simulink model "Experiment_1_cs"  (Simulink 8.4)
settings: Solver=ode5  SolverMode=SingleTasking  StartTime=0.0  StopTime=inf  FixedStep=1/100  RelTol=1e-3
PreLoadFcn:
  | mbxruntime.callbacks.PreLoadFcn(bdroot);
PostLoadFcn:
  | mbxruntime.callbacks.PostLoadFcn(bdroot);
InitFcn:
  | mbxruntime.callbacks.InitFcn(bdroot);
StartFcn:
  | mbxruntime.callbacks.StartFcn(bdroot);
StopFcn:
  | mbxruntime.callbacks.StopFcn(bdroot);
undefined symbols (not defined in the file or in its folder): dfreq, gray, Rec, SDTV, strel
libraries: simulink x42, PreScanSimulinkLibrary x17, visiontextngfix x15, simulink_extras x12, visionconversions x3, PreScanUsefulBlocks x3, visionsinks x2, visionstatistics x1, visionmorphops x1, visionanalysis x1, simulink_need_slupdate x1
(part 2 of 8)

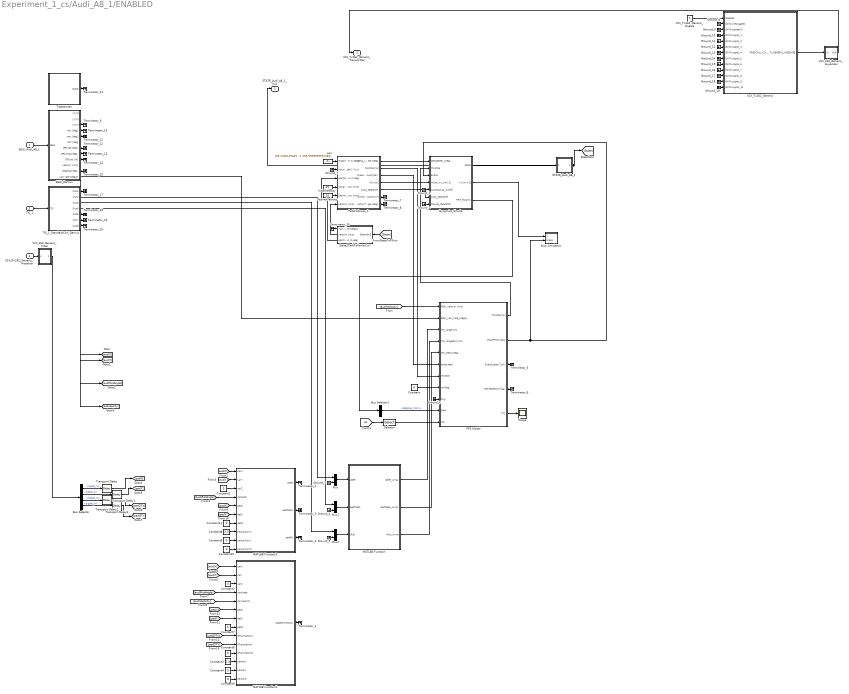
== system Experiment_1_cs/Audi_A8_1/ENABLED ==
  SELF_Audi_A8_1 : Inport  Tag=inport/SelfPort  OutDataTypeStr=Bus: PRESCAN_SELFSENSORDATA  PortDimensions=1  SampleTime=1/100  BusOutputAsStruct=on
  TIS_1 : Inport  Tag=inport/TIS  Port=2  OutDataTypeStr=Bus: PRESCAN_SCANNERSENSOR_MESSAGE  PortDimensions=1  SampleTime=1/50  BusOutputAsStruct=on
  V2X_Rx262_Generic_Receiver : Inport  Tag=inport/plugin/sfun_V2X_Generic_Receiver  Port=3  BusOutputAsStruct=on
  Bus Selector : BusSelector  OutputSignals=DATA.signal_1,DATA.signal_2,DATA.signal_3,DATA.signal_4
  Bus Selector1 : BusSelector  OutputSignals=NEngine_[rpm]
  Constant{,1..2,4..7,9..11} (10 alike) : Constant  Value=0
  Constant3 : Constant  Value=2.3
  Constant8 : Constant  Value=2.3
  DesiredVelocity : Constant  Tag=DesiredVelocity  Value=15
  Dynamics_Simple : Subsystem  Tag=Simple_Vehicle_Dynamics  mask(PreScan Block: Simple Dynamics){Migrate=on, TimeStep=1/100, ComputationMode=Continuous_Time}
      mask prompts: Migrate "Migrate. During migration this block will be replaced by a newer one."; TimeStep "Auto assigned: Time Step [s]"; ComputationMode "Computation mode:"
      mask help:
      | The Simple Dynamics Model is selected in the GUI to simulate vehicle dynamics behavior.
      |
      | The Simple Dynamics Model is completely open to the user. The parameters of this model can be set in the Simple Dynamics dialog in the GUI.
      |
      | For more information, please click Help.
      mask init:
      | p = SimpleDyn_pars;
      settings: DeleteFcn=PreScanBlockDeleteFcn;
      mask Help: eval('openHelp(220)')
      mask Display:
      | image(imread('SimpleDyn.png'))
      | port_label('input', 1, '{\delta}_S_t_ _e_e_r [deg]','texmode','on')
      | port_label('input', 2, 'Throttle [%]')
      | port_label('input', 3, 'Brake Pres [bar]')
      | port_label('input', 4, 'V_0 [ms-1]','texmode','on')
      | port_label('input', 5, 'Auto=[0]/Manual=[1]')
      | port_label('input', 6, 'Auto_GearShift')
      | port_label('input', 7, 'Manual_GearShift')
      | port_label('output', 1, 'State')
      | port_label('output', 2, 'Vx [ms-1]')
      | port_label('output', 3, 'Perf Params')
  Ground_{1..19} (19 alike) : Ground
  InitialVelocity : Constant  Tag=InitialVelocity  Value=15
  MATLAB Function : MATLAB Function  TreatAsAtomicUnit=on
  MATLAB Function1 : MATLAB Function  TreatAsAtomicUnit=on
  MATLAB Function2 : MATLAB Function  TreatAsAtomicUnit=on
  Mux : Mux  Inputs=2
  Mux1 : Mux  Inputs=2
  Mux2 : Mux  Inputs=2
  PPS Model : Subsystem  mask(PPS Model){MaxSpeed=70, MaxBrakePressure=150, BrakeDelay=100, LaneWidth=3.5, TISMaxRange=40, TISMaxTheta=60, TISfreq=25, TISdet=32, Camfreq=50, Mainfreq=100, DisplaySwitch=on, DisplayFreq=25, RadarSwitch=on, RadarFreq=25}
      mask prompts: MaxSpeed "Vehicle cut-off speed [km/h]"; MaxBrakePressure "Maximum value of braking pressure available [bar]"; BrakeDelay "Braking system delay [ms]"; LaneWidth "Lane width [m]"; TISMaxRange "TIS maximum range [m]"; TISMaxTheta "TIS maximum theta [deg]"; TISfreq "TIS frequency [Hz]"; TISdet "Max. number of Radar detected objects [-]"; Camfreq "Camera frequency [Hz]"; Mainfreq "Compilation sheet frequency [Hz]"; DisplaySwitch "Show EGO parameters visualization"; DisplayFreq "EGO parameters visualization frequency [Hz]"; RadarSwitch "Show radar visualization"; RadarFreq "Radar frequency [Hz]"
      mask help: PreScan Experiment and Pedestrian Protection System parameters
      mask Help: eval('openHelp(8130)')
      mask Callback DisplaySwitch:
      | en = get_param(gcb,'MaskEnables');
      | switch get_param(gcb, 'DisplaySwitch')
      |     case 'off'
      |         en{12} = 'off';
      |     case 'on'
      |         en{12} = 'on';
      | end
      | set_param(gcb,'MaskEnables',en);
      mask Callback RadarSwitch:
      | en = get_param(gcb,'MaskEnables');
      | switch get_param(gcb, 'RadarSwitch')
      |     case 'off'
      |         en{14} = 'off';
      |     case 'on'
      |         en{14} = 'on';
      | end
      | set_param(gcb,'MaskEnables',en);
  PathFollower_1 : Subsystem  Tag=pathFollower  mask(PreScan Block: Path Follower){Migrate=on, FileName='Trajectory_2.mat', TunableSteeringGain=1, XShifting_wrt_COG=0}
      mask prompts: Migrate "Migrate. During migration this block will be replaced by a newer one."; FileName "Trajectory Name"; TunableSteeringGain "TunableSteeringGain [-]"; XShifting_wrt_COG "XShifting_wrt_COG [m]"
      mask help:
      | The Path Follower Model is selected in the GUI to simulate driver behavior.
      |
      | For more information, please click Help.
      mask init:
      | load(['trajectories/',eval(FileName)])
      | traject=trajectory';
      | 
      | Traj_x=traject(:,2);
      | Traj_y=traject(:,3);
      | Traj_z=traject(:,4);
      | Traj_vx=traject(:,8);
      | Traj_vy=traject(:,9);
      | Traj_vz=traject(:,10);
      mask Help: eval('openHelp(232)')
  SELF_Demux : Subsystem  Tag=demux/SelfPort  mask(PreScan Demux Block:){}
      mask help:
      | The SELF port shows (state) information of the actor itself. The outputs are position in the experiment's axis system and the GPS coordinates, and the object's absolute velocity and compass heading.
      |
      | For more information, please click Help.
      settings: DeleteFcn=PreScanBlockDeleteFcn;
      mask Help: eval('openHelp(462)')
      mask Display:
      | port_label('output',1,'x [m]')
      | port_label('output',2,'y [m]')
      | port_label('output',3,'z [m]','texmode','on')
      | port_label('output',4,'Rotx [deg]','texmode','on')
      | port_label('output',5,'Roty [deg]','texmode','on')
      | port_label('output',6,'Rotz [deg]','texmode','on')
      | port_label('output',7,'GPS lat [deg]','texmode','on')
      | port_label('output',8,'GPS long [deg]','texmode','on')
      | port_label('output',9,'GPS alt [m]','texmode','on')
      | port_label('output',10,'Velocity [m/s]')
      | port_label('output',11,'Heading [deg]')
      | port_label('output',12,'Yaw rate [deg/s]')
  STATE_Audi_A8_1 : Subsystem  Tag=mux/StatePort  Priority=0  LoadFcn=load PrescanStateActuatorData  mask(PreScan Sink Block: State){x0=99.430015563964844, y0=124.71636199951172, z0=0.55, Roll0=0, Pitch0=0, Yaw0=359.9999999997284, TimeStep=1/100}
      mask prompts: x0 "Ini x-position VEHICLE wrt GLOBAL axis system [m]"; y0 "Ini y-position VEHICLE wrt GLOBAL axis system [m]"; z0 "Ini z-position VEHICLE wrt GLOBAL axis system [m]"; Roll0 "Ini roll-angle BODY wrt VEHICLE axis system [deg]"; Pitch0 "Ini pitch-angle BODY wrt VEHICLE axis system [deg]"; Yaw0 "Ini yaw-angle VEHICLE wrt GLOBAL axis system [deg]"; TimeStep "Auto-Assigned: Upload Period [s]"
      mask help:
      | The Actor State contains a vector signal of size (9x1), containing the following signals:
      |
      | -  Position                  (x,y,z)                                     [m]
      | -  Velocity                  (vx,vy,vz)                               [m/s]
      | -  Angles                    (Roll, Pitch, Yaw)                   [rad]
      |
      | The Actor state is defined in the global axis system.
      | The state is superponed on the Initial position defined in the GUI.
      |
      | For more information, please click Help.
      settings: DeleteFcn=PreScanBlockDeleteFcn;
      mask Help: eval('openHelp(222)')
      mask Display: image(imread('State.png'))
  Scope : Scope
  Selector : Selector  InputPortWidth=5
  State2PathFollowerCnv : Subsystem  Tag=State2PFConnection/cnv
  Stop simulation : Subsystem
  TIS_1_StandardCoh_Demux : Subsystem  Tag=demux/TIS/StandardCoh  TreatAsAtomicUnit=on  mask(PreScan Demux Block: TIS){MAXMESSAGES=1}
      mask prompts: MAXMESSAGES "Number of Objects"
      mask Help: eval('openHelp(449)')
      mask Display:
      | port_label('input',1,'TIS')
      | port_label('output',1,'Beam ID [-]')
      | port_label('output',2,'Range [m]')
      | port_label('output',3,'DopplerVelocity [m/s]')
      | port_label('output',4,'{\theta} [deg]','texmode','on')
      | port_label('output',5,'{\phi} [deg]','texmode','on')
      | port_label('output',6,'Target ID [-]','texmode','on')
      | port_label('output',7,'TIS Data','texmode','on')
  Terminator_{1..21} (21 alike) : Terminator
  Trajectories : Subsystem  Tag=Trajectories  mask(PreScan Source Block: Trajectories){}
      mask help:
      | The Trajectory block contains the trajectories defined in the PreScan Experiment Editor. The output of the trajectory block is the (vehicle) State.
      |
      | For more information, please click Help.
      settings: DeleteFcn=PreScanBlockDeleteFcn;
      mask Help: eval('openHelp(312)')
      mask Display: image(imread('Trajectory.png'));
  Transport Delay{,1..3} (4 alike) : TransportDelay  DelayTime=0
  V2X_262_Generic_Expander : Subsystem  LoadFcn=addpath .\V2XPlugin; V2Xbusses;
  V2X_262_Generic_Filter : Subsystem
      mask Display: disp('[1]');
  V2X_Tx262_Generic : Subsystem
  V2X_Tx262_Generic_Enable : Constant  OutDataTypeStr=Inherit: Inherit via back propagation
  pos : Constant  Tag=pos  Value=[99.430015563964844 124.71636199951172 359.9999999997284]
  STATE_Audi_A8_1_bus : Outport  Tag=outport/StatePort  OutDataTypeStr=Bus: PRESCAN_STATEACTUATORDATA  PortDimensions=1  SampleTime=1/100
  V2X_Tx262_Generic_Transmitter : Outport  Tag=outport/plugin/sfun_V2X_Generic_Transmitter  Port=2
  wires:
  Dynamics_Simple/3(Perf_Params) -> Bus Selector1/1
  SELF_Demux/12(yaw rate [deg/s]) -> PPS Model/2(EGO_yaw_rate_[deg/s])
  TIS_1_StandardCoh_Demux/2(Out2) -> Mux/1
  TIS_1_StandardCoh_Demux/3(Out3) -> Mux2/1
  TIS_1_StandardCoh_Demux/4(Out4) -> Mux1/1
  [audiX] -> MATLAB Function2/1(carX)
  [audiY] -> MATLAB Function2/2(carY)
  Constant1/1 -> MATLAB Function2/3(carZ)
  [audiRotAngle] -> MATLAB Function2/4(carRotZ)
  [audiX] -> MATLAB Function1/1(carX)
  [audiY] -> MATLAB Function1/2(carY)
  Constant2/1 -> MATLAB Function1/3(carZ)
  [audiRotAngle] -> MATLAB Function1/4(carAngle)
  [audiVelocity] -> MATLAB Function1/5(carVelocity)
  Constant3/1 -> MATLAB Function1/12(sensorX)
  Constant4/1 -> MATLAB Function1/13(sensorY)
  Constant5/1 -> MATLAB Function1/14(sensorZ)
  Constant6/1 -> MATLAB Function1/11(dTranslationZ)
  Constant7/1 -> MATLAB Function1/8(pedZ)
  Constant8/1 -> MATLAB Function2/8(sensorCorrX)
  Constant9/1 -> MATLAB Function2/9(sensorCorrY)
  Constant10/1 -> MATLAB Function2/10(sensorCorrZ)
  Constant11/1 -> MATLAB Function2/7(pedZ)
  [pedX] -> MATLAB Function2/5(pedX)
  [pedY] -> MATLAB Function2/6(pedY)
  [pedX] -> MATLAB Function1/6(pedX)
  [pedY] -> MATLAB Function1/7(pedY)
  [pedDTX] -> MATLAB Function1/9(dTranslationX)
  [pedDTY] -> MATLAB Function1/10(dTranslationY)
  SELF_Demux/1(x [m]) -> [audiX]
  SELF_Demux/2(y [m]) -> [audiY]
  SELF_Demux/6(rotz [deg]) -> [audiRotAngle]
  SELF_Demux/10(velocity [m/s]) -> [audiVelocity]
  [audiVelocity] -> PPS Model/1(EGO_velocity [m/s])
  Bus Selector1/1 -> PPS Model/10(RPM)  "<NEngine_[rpm]>"
  [cd] -> Selector/1
  PPS Model/1(Throttle [%]) -> Dynamics_Simple/2(Throttle)
  PPS Model/2(BrakePres [bar]) -> Dynamics_Simple/3(Brake), Stop simulation/2(brake)
  Bus Selector/1 -> Transport Delay/1  "<signal_1>"
  Bus Selector/2 -> Transport Delay1/1  "<signal_2>"
  Bus Selector/3 -> Transport Delay2/1  "<signal_3>"
  Bus Selector/4 -> Transport Delay3/1  "<signal_4>"
  Mux/1 -> MATLAB Function/1(pedR)
  Mux1/1 -> MATLAB Function/2(pedTheta)
  Mux2/1 -> MATLAB Function/3(dVel)
  Dynamics_Simple/2(Vx [m s-1]) -> Stop simulation/1(V)
  V2X_262_Generic_Filter/1(Filter_Out) -> Bus Selector/1
  Transport Delay/1 -> [pedX]
  Transport Delay1/1 -> [pedY]
  Transport Delay2/1 -> [pedDTX]
  Transport Delay3/1 -> [pedDTY]
  PPS Model/5(TTC) -> Scope/1
  Selector/1 -> PPS Model/11(CD)
  PathFollower_1/2(throttle [%]) -> PPS Model/7(throttle)
  PathFollower_1/3(brake pressure [bar]) -> PPS Model/6(brake dem)
  Constant/1 -> PPS Model/8(ind flag)
  MATLAB Function/1(pedR_Array) -> PPS Model/3(TIS_range [m])
  MATLAB Function/2(pedTheta_Array) -> PPS Model/5(TIS_theta [deg])
  MATLAB Function/3(dVel_Array) -> PPS Model/4(TIS_rangedot [m/s])
  STATE_Audi_A8_1/1(StateBus) -> STATE_Audi_A8_1_bus/1, [State]
  SELF_Audi_A8_1/1 -> SELF_Demux/1(SELF)
  TIS_1/1 -> TIS_1_StandardCoh_Demux/1(TIS)
  pos/1 -> PathFollower_1/1(TrajOffset_x,y,Y [m,m,deg])
  InitialVelocity/1 -> PathFollower_1/4(Initial Velocity [m/s])
  DesiredVelocity/1 -> PathFollower_1/5(Desired Velocity [m/s])
  [State] -> State2PathFollowerCnv/1(State BUS)
  State2PathFollowerCnv/2(velocity [m/s]) -> PathFollower_1/6(velocity [m/s])
  State2PathFollowerCnv/3(position x,y,Y [m,m,deg]) -> PathFollower_1/3(position x,y,Y [m,m,deg])
  PathFollower_1/1(delta_steerwheel [deg]) -> Dynamics_Simple/1(DeltaSteer_[deg])
  PathFollower_1/4(v0 [m/s]) -> Dynamics_Simple/4(Initial_Vx_[ms-1])
  PathFollower_1/5(Auto_GearShift) -> Dynamics_Simple/6(Auto_GearShift)
  Dynamics_Simple/1(State) -> STATE_Audi_A8_1/1(State)
  V2X_Tx262_Generic_Enable/1 -> V2X_Tx262_Generic/1(Enabled)
  V2X_Tx262_Generic/1(PRESCAN_V2X_USER_GENERIC_MESSAGE) -> V2X_262_Generic_Expander/1(In)
  V2X_262_Generic_Expander/1(Out) -> V2X_Tx262_Generic_Transmitter/1
  V2X_Rx262_Generic_Receiver/1 -> V2X_262_Generic_Filter/1(Filter_In)
  Ground_1/1 -> Dynamics_Simple/5(AutoManual_OnOff)
  Ground_2/1 -> Dynamics_Simple/7(Manual_GearShift)
  MATLAB Function1/1(dopplerVelocity) -> Terminator_1/1
  MATLAB Function2/1(pedR) -> Terminator_2/1
  MATLAB Function2/2(pedTheta) -> Terminator_3/1
  MATLAB Function2/3(pedPhi) -> Terminator_4/1
  Ground_3/1 -> Mux/2
  Ground_4/1 -> Mux1/2
  Ground_5/1 -> Mux2/2
  Ground_6/1 -> PPS Model/9(img)
  PPS Model/3(BrakeLights (3x1)) -> Terminator_5/1
  PPS Model/4(Ped detection flag) -> Terminator_6/1
  Ground_7/1 -> PathFollower_1/2(ActorOffset_Left(+) / Right(-) [m])
  PathFollower_1/6(Actor/Traj_distance [m]) -> Terminator_7/1
  PathFollower_1/7(Actor/Traj_angle [deg]) -> Terminator_8/1
  SELF_Demux/3(z [m]) -> Terminator_9/1
  SELF_Demux/4(rotx [deg]) -> Terminator_10/1
  SELF_Demux/5(roty [deg]) -> Terminator_11/1
  SELF_Demux/7(GPS lat [deg]) -> Terminator_12/1
  SELF_Demux/8(GPS long [deg]) -> Terminator_13/1
  SELF_Demux/9(GPS alt [m]) -> Terminator_14/1
  SELF_Demux/11(heading [deg]) -> Terminator_15/1
  State2PathFollowerCnv/1(Yaw rate [deg/s]) -> Terminator_16/1
  TIS_1_StandardCoh_Demux/1(Out1) -> Terminator_17/1
  TIS_1_StandardCoh_Demux/5(Out5) -> Terminator_18/1
  TIS_1_StandardCoh_Demux/6(Out7) -> Terminator_19/1
  TIS_1_StandardCoh_Demux/7(Out6) -> Terminator_20/1
  Trajectories/1(State) -> Terminator_21/1
  Ground_8/1 -> V2X_Tx262_Generic/2(DATA.messageID)
  Ground_9/1 -> V2X_Tx262_Generic/3(DATA.senderID)
  Ground_10/1 -> V2X_Tx262_Generic/4(DATA.signal_1)
  Ground_11/1 -> V2X_Tx262_Generic/5(DATA.signal_2)
  Ground_12/1 -> V2X_Tx262_Generic/6(DATA.signal_3)
  Ground_13/1 -> V2X_Tx262_Generic/7(DATA.signal_4)
  Ground_14/1 -> V2X_Tx262_Generic/8(DATA.signal_5)
  Ground_15/1 -> V2X_Tx262_Generic/9(DATA.signal_6)
  Ground_16/1 -> V2X_Tx262_Generic/10(DATA.signal_7)
  Ground_17/1 -> V2X_Tx262_Generic/11(DATA.signal_8)
  Ground_18/1 -> V2X_Tx262_Generic/12(DATA.signal_9)
  Ground_19/1 -> V2X_Tx262_Generic/13(DATA.signal_10)

== system Experiment_1_cs/BMW_Z3_1/DISABLED ==
  SELF_BMW_Z3_1 : Inport  Tag=inport/SelfPort  OutDataTypeStr=Bus: PRESCAN_SELFSENSORDATA  PortDimensions=1  SampleTime=1/100  BusOutputAsStruct=on
  TIS_2 : Inport  Tag=inport/TIS  Port=2  OutDataTypeStr=Bus: PRESCAN_SCANNERSENSOR_MESSAGE  PortDimensions=1  SampleTime=1/50  BusOutputAsStruct=on
  V2X_Rx264_Generic_Receiver : Inport  Tag=inport/plugin/sfun_V2X_Generic_Receiver  Port=3  BusOutputAsStruct=on
  GND1 : Subsystem
  GND2 : Ground
  TRM1 : Terminator
  TRM2 : Terminator
  TRM3 : Terminator
  STATE_BMW_Z3_1_bus : Outport  Tag=outport/StatePort  OutDataTypeStr=Bus: PRESCAN_STATEACTUATORDATA  PortDimensions=1  SampleTime=1/100
  V2X_Tx264_Generic_Transmitter : Outport  Tag=outport/plugin/sfun_V2X_Generic_Transmitter  Port=2
  wires:
  SELF_BMW_Z3_1/1 -> TRM1/1
  TIS_2/1 -> TRM2/1
  V2X_Rx264_Generic_Receiver/1 -> TRM3/1
  GND1/1(bus) -> STATE_BMW_Z3_1_bus/1
  GND2/1 -> V2X_Tx264_Generic_Transmitter/1

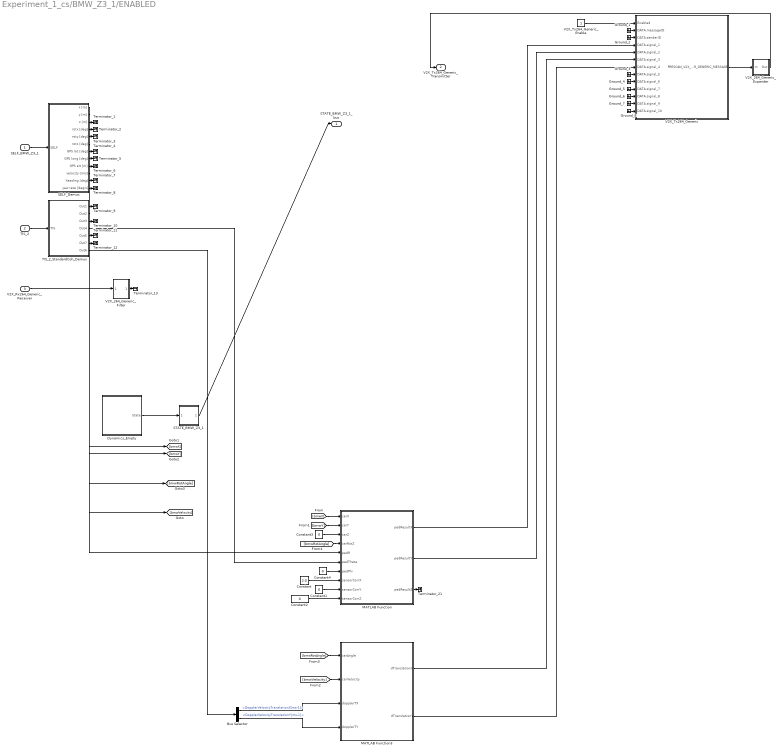
== system Experiment_1_cs/BMW_Z3_1/ENABLED ==
  SELF_BMW_Z3_1 : Inport  Tag=inport/SelfPort  OutDataTypeStr=Bus: PRESCAN_SELFSENSORDATA  PortDimensions=1  SampleTime=1/100  BusOutputAsStruct=on
  TIS_2 : Inport  Tag=inport/TIS  Port=2  OutDataTypeStr=Bus: PRESCAN_SCANNERSENSOR_MESSAGE  PortDimensions=1  SampleTime=1/50  BusOutputAsStruct=on
  V2X_Rx264_Generic_Receiver : Inport  Tag=inport/plugin/sfun_V2X_Generic_Receiver  Port=3  BusOutputAsStruct=on
  Bus Selector : BusSelector  OutputSignals=DopplerVelocityTranslationX[ms-1],DopplerVelocityTranslationY[ms-1]
  Constant : Constant  Value=2.0
  Constant{1..4} (4 alike) : Constant  Value=0
  Dynamics_Empty : Subsystem  Tag=Dynamics_Empty
      mask Help: eval('openHelp(202)')
      mask Display: port_label('output', 1, 'State');text(0,0,' Empty\n')
  Ground_{1..8} (8 alike) : Ground
  MATLAB Function : MATLAB Function  TreatAsAtomicUnit=on
  MATLAB Function3 : MATLAB Function  TreatAsAtomicUnit=on
  SELF_Demux : Subsystem  Tag=demux/SelfPort  mask(PreScan Demux Block:){}
      mask help:
      | The SELF port shows (state) information of the actor itself. The outputs are position in the experiment's axis system and the GPS coordinates, and the object's absolute velocity and compass heading.
      |
      | For more information, please click Help.
      settings: DeleteFcn=PreScanBlockDeleteFcn;
      mask Help: eval('openHelp(462)')
      mask Display:
      | port_label('output',1,'x [m]')
      | port_label('output',2,'y [m]')
      | port_label('output',3,'z [m]','texmode','on')
      | port_label('output',4,'Rotx [deg]','texmode','on')
      | port_label('output',5,'Roty [deg]','texmode','on')
      | port_label('output',6,'Rotz [deg]','texmode','on')
      | port_label('output',7,'GPS lat [deg]','texmode','on')
      | port_label('output',8,'GPS long [deg]','texmode','on')
      | port_label('output',9,'GPS alt [m]','texmode','on')
      | port_label('output',10,'Velocity [m/s]')
      | port_label('output',11,'Heading [deg]')
      | port_label('output',12,'Yaw rate [deg/s]')
  STATE_BMW_Z3_1 : Subsystem  Tag=mux/StatePort  Priority=0  LoadFcn=load PrescanStateActuatorData  mask(PreScan Sink Block: State){x0=157.54670715332031, y0=142.41622924804687, z0=0.4784, Roll0=0, Pitch0=0, Yaw0=270, TimeStep=1/100}
      mask prompts: x0 "Ini x-position VEHICLE wrt GLOBAL axis system [m]"; y0 "Ini y-position VEHICLE wrt GLOBAL axis system [m]"; z0 "Ini z-position VEHICLE wrt GLOBAL axis system [m]"; Roll0 "Ini roll-angle BODY wrt VEHICLE axis system [deg]"; Pitch0 "Ini pitch-angle BODY wrt VEHICLE axis system [deg]"; Yaw0 "Ini yaw-angle VEHICLE wrt GLOBAL axis system [deg]"; TimeStep "Auto-Assigned: Upload Period [s]"
      mask help:
      | The Actor State contains a vector signal of size (9x1), containing the following signals:
      |
      | -  Position                  (x,y,z)                                     [m]
      | -  Velocity                  (vx,vy,vz)                               [m/s]
      | -  Angles                    (Roll, Pitch, Yaw)                   [rad]
      |
      | The Actor state is defined in the global axis system.
      | The state is superponed on the Initial position defined in the GUI.
      |
      | For more information, please click Help.
      settings: DeleteFcn=PreScanBlockDeleteFcn;
      mask Help: eval('openHelp(222)')
      mask Display: image(imread('State.png'))
  TIS_2_StandardCoh_Demux : Subsystem  Tag=demux/TIS/StandardCoh  TreatAsAtomicUnit=on  mask(PreScan Demux Block: TIS){MAXMESSAGES=1}
      mask prompts: MAXMESSAGES "Number of Objects"
      mask Help: eval('openHelp(449)')
      mask Display:
      | port_label('input',1,'TIS')
      | port_label('output',1,'Beam ID [-]')
      | port_label('output',2,'Range [m]')
      | port_label('output',3,'DopplerVelocity [m/s]')
      | port_label('output',4,'{\theta} [deg]','texmode','on')
      | port_label('output',5,'{\phi} [deg]','texmode','on')
      | port_label('output',6,'Target ID [-]','texmode','on')
      | port_label('output',7,'TIS Data','texmode','on')
  Terminator_{1..13,21} (14 alike) : Terminator
  V2X_264_Generic_Expander : Subsystem  LoadFcn=addpath .\V2XPlugin; V2Xbusses;
  V2X_264_Generic_Filter : Subsystem
      mask Display: disp('[1]');
  V2X_Tx264_Generic : Subsystem
  V2X_Tx264_Generic_Enable : Constant  OutDataTypeStr=Inherit: Inherit via back propagation
  STATE_BMW_Z3_1_bus : Outport  Tag=outport/StatePort  OutDataTypeStr=Bus: PRESCAN_STATEACTUATORDATA  PortDimensions=1  SampleTime=1/100
  V2X_Tx264_Generic_Transmitter : Outport  Tag=outport/plugin/sfun_V2X_Generic_Transmitter  Port=2
  wires:
  SELF_Demux/1(x [m]) -> [bmwX]
  SELF_Demux/2(y [m]) -> [bmwY]
  SELF_Demux/6(rotz [deg]) -> [bmwRotAngle]
  SELF_Demux/10(velocity [m/s]) -> [bmwVelocity]
  TIS_2_StandardCoh_Demux/2(Out2) -> MATLAB Function/5(pedR)
  TIS_2_StandardCoh_Demux/4(Out4) -> MATLAB Function/6(pedTheta)
  TIS_2_StandardCoh_Demux/7(Out6) -> Bus Selector/1
  MATLAB Function/1(pedResultX) -> V2X_Tx264_Generic/4(DATA.signal_1)
  MATLAB Function/2(pedResultY) -> V2X_Tx264_Generic/5(DATA.signal_2)
  MATLAB Function3/1(dTranslationX) -> V2X_Tx264_Generic/6(DATA.signal_3)
  MATLAB Function3/2(dTranslationY) -> V2X_Tx264_Generic/7(DATA.signal_4)
  Constant/1 -> MATLAB Function/8(sensorCorrX)
  Constant1/1 -> MATLAB Function/9(sensorCorrY)
  Constant2/1 -> MATLAB Function/10(sensorCorrZ)
  Constant3/1 -> MATLAB Function/3(carZ)
  Constant4/1 -> MATLAB Function/7(pedPhi)
  Bus Selector/1 -> MATLAB Function3/3(dopplerTX)  "<DopplerVelocityTranslationX[ms-1]>"
  Bus Selector/2 -> MATLAB Function3/4(dopplerTY)  "<DopplerVelocityTranslationY[ms-1]>"
  [bmwX] -> MATLAB Function/1(carX)
  [bmwY] -> MATLAB Function/2(carY)
  [bmwVelocity] -> MATLAB Function3/2(carVelocity)
  [bmwRotAngle] -> MATLAB Function3/1(carAngle)
  [bmwRotAngle] -> MATLAB Function/4(carRotZ)
  MATLAB Function/3(pedResultZ) -> Terminator_21/1
  STATE_BMW_Z3_1/1(StateBus) -> STATE_BMW_Z3_1_bus/1
  SELF_BMW_Z3_1/1 -> SELF_Demux/1(SELF)
  TIS_2/1 -> TIS_2_StandardCoh_Demux/1(TIS)
  Dynamics_Empty/1(State) -> STATE_BMW_Z3_1/1(State)
  V2X_Tx264_Generic_Enable/1 -> V2X_Tx264_Generic/1(Enabled)
  V2X_Tx264_Generic/1(PRESCAN_V2X_USER_GENERIC_MESSAGE) -> V2X_264_Generic_Expander/1(In)
  V2X_264_Generic_Expander/1(Out) -> V2X_Tx264_Generic_Transmitter/1
  V2X_Rx264_Generic_Receiver/1 -> V2X_264_Generic_Filter/1(Filter_In)
  SELF_Demux/3(z [m]) -> Terminator_1/1
  SELF_Demux/4(rotx [deg]) -> Terminator_2/1
  SELF_Demux/5(roty [deg]) -> Terminator_3/1
  SELF_Demux/7(GPS lat [deg]) -> Terminator_4/1
  SELF_Demux/8(GPS long [deg]) -> Terminator_5/1
  SELF_Demux/9(GPS alt [m]) -> Terminator_6/1
  SELF_Demux/11(heading [deg]) -> Terminator_7/1
  SELF_Demux/12(yaw rate [deg/s]) -> Terminator_8/1
  TIS_2_StandardCoh_Demux/1(Out1) -> Terminator_9/1
  TIS_2_StandardCoh_Demux/3(Out3) -> Terminator_10/1
  TIS_2_StandardCoh_Demux/5(Out5) -> Terminator_11/1
  TIS_2_StandardCoh_Demux/6(Out7) -> Terminator_12/1
  V2X_264_Generic_Filter/1(Filter_Out) -> Terminator_13/1
  Ground_1/1 -> V2X_Tx264_Generic/2(DATA.messageID)
  Ground_2/1 -> V2X_Tx264_Generic/3(DATA.senderID)
  Ground_3/1 -> V2X_Tx264_Generic/8(DATA.signal_5)
  Ground_4/1 -> V2X_Tx264_Generic/9(DATA.signal_6)
  Ground_5/1 -> V2X_Tx264_Generic/10(DATA.signal_7)
  Ground_6/1 -> V2X_Tx264_Generic/11(DATA.signal_8)
  Ground_7/1 -> V2X_Tx264_Generic/12(DATA.signal_9)
  Ground_8/1 -> V2X_Tx264_Generic/13(DATA.signal_10)

== system Experiment_1_cs/CollisionDetection/DISABLED ==
  GND1 : Subsystem
  CollisionDetection : Outport  Tag=outport/CollisionDetection  OutDataTypeStr=Bus: PRESCAN_COLLISIONDETECTION_MESSAGE  PortDimensions=5  SampleTime=1/100
  wires:
  GND1/1(bus) -> CollisionDetection/1

== system Experiment_1_cs/CollisionDetection/ENABLED ==
  Sensor : S-Function  FunctionName=sfun_CollisionDetection  Parameters=detectableCollisions, timestep  EnableBusSupport=off  mask(PreScan Source Block: CollisionDetection){detectableCollisions=5, timestep=1/100}
      mask prompts: detectableCollisions "Max detectable collisions:"; timestep "MATLAB timestep:"
      mask help: Collision Detection can be used to detect collisions between PreScan components. For Collision Detection the actual component shape is taken into account, so it is not a bounding box approach.
      mask Help: eval('openHelp(811)')
      mask Display: image(imread('crash.jpg'))
  CollisionDetection : Outport  Tag=outport/CollisionDetection  OutDataTypeStr=Bus: PRESCAN_COLLISIONDETECTION_MESSAGE  PortDimensions=5  SampleTime=1/100
  wires:
  Sensor/1 -> CollisionDetection/1

== system Experiment_1_cs/Male_RegularAni_1/DISABLED ==
  SELF_Male_RegularAni_1 : Inport  Tag=inport/SelfPort  OutDataTypeStr=Bus: PRESCAN_SELFSENSORDATA  PortDimensions=1  SampleTime=1/100  BusOutputAsStruct=on
  GND1 : Subsystem
  GND2 : Subsystem
  TRM1 : Terminator
  STATE_Male_RegularAni_1_bus : Outport  Tag=outport/StatePort  OutDataTypeStr=Bus: PRESCAN_STATEACTUATORDATA  PortDimensions=1  SampleTime=1/100
  ANIM_Male_RegularAni_1 : Outport  Tag=outport/AnimationOutport  Port=2  OutDataTypeStr=Bus: PRESCAN_ANIMACTUATORDATA  PortDimensions=1  SampleTime=1/100
  wires:
  SELF_Male_RegularAni_1/1 -> TRM1/1
  GND1/1(bus) -> STATE_Male_RegularAni_1_bus/1
  GND2/1(bus) -> ANIM_Male_RegularAni_1/1

== system Experiment_1_cs/Male_RegularAni_1/ENABLED ==
  SELF_Male_RegularAni_1 : Inport  Tag=inport/SelfPort  OutDataTypeStr=Bus: PRESCAN_SELFSENSORDATA  PortDimensions=1  SampleTime=1/100  BusOutputAsStruct=on
  Animation : Subsystem  Tag=RunningHumanAnimation  mask(Prescan Conversion Block: Running Human Animation){MWS=1.95, WalkingScale=1.0, RunningScale=1.0, TimeStep=1/100}
      mask prompts: MWS "Maximum Walking Speed [m/s], above which the animation will switch to running mode."; WalkingScale "Walking mode scaling factor to sync the animation frames to the displacement."; RunningScale "Running mode scaling factor to sync the animation frames to the displacement."; TimeStep "Auto-Assigned: Upload Period [s]"
      mask help: The Running Human Animation block converts the State signal of a human into signals to properly control the animation.
      mask Help: eval('openHelp(239)');
      mask Display: image(imread('HumanAnimated.jpg'))
  SELF_Demux : Subsystem  Tag=demux/SelfPort  mask(PreScan Demux Block:){}
      mask help:
      | The SELF port shows (state) information of the actor itself. The outputs are position in the experiment's axis system and the GPS coordinates, and the object's absolute velocity and compass heading.
      |
      | For more information, please click Help.
      settings: DeleteFcn=PreScanBlockDeleteFcn;
      mask Help: eval('openHelp(462)')
      mask Display:
      | port_label('output',1,'x [m]')
      | port_label('output',2,'y [m]')
      | port_label('output',3,'z [m]','texmode','on')
      | port_label('output',4,'Rotx [deg]','texmode','on')
      | port_label('output',5,'Roty [deg]','texmode','on')
      | port_label('output',6,'Rotz [deg]','texmode','on')
      | port_label('output',7,'GPS lat [deg]','texmode','on')
      | port_label('output',8,'GPS long [deg]','texmode','on')
      | port_label('output',9,'GPS alt [m]','texmode','on')
      | port_label('output',10,'Velocity [m/s]')
      | port_label('output',11,'Heading [deg]')
      | port_label('output',12,'Yaw rate [deg/s]')
  STATE_Male_RegularAni_1 : Subsystem  Tag=mux/StatePort  Priority=0  LoadFcn=load PrescanStateActuatorData  mask(PreScan Sink Block: State){x0=150.46946716308594, y0=129.23065948486328, z0=0, Roll0=0, Pitch0=0, Yaw0=269.97511419716352, TimeStep=1/100}
      mask prompts: x0 "Ini x-position VEHICLE wrt GLOBAL axis system [m]"; y0 "Ini y-position VEHICLE wrt GLOBAL axis system [m]"; z0 "Ini z-position VEHICLE wrt GLOBAL axis system [m]"; Roll0 "Ini roll-angle BODY wrt VEHICLE axis system [deg]"; Pitch0 "Ini pitch-angle BODY wrt VEHICLE axis system [deg]"; Yaw0 "Ini yaw-angle VEHICLE wrt GLOBAL axis system [deg]"; TimeStep "Auto-Assigned: Upload Period [s]"
      mask help:
      | The Actor State contains a vector signal of size (9x1), containing the following signals:
      |
      | -  Position                  (x,y,z)                                     [m]
      | -  Velocity                  (vx,vy,vz)                               [m/s]
      | -  Angles                    (Roll, Pitch, Yaw)                   [rad]
      |
      | The Actor state is defined in the global axis system.
      | The state is superponed on the Initial position defined in the GUI.
      |
      | For more information, please click Help.
      settings: DeleteFcn=PreScanBlockDeleteFcn;
      mask Help: eval('openHelp(222)')
      mask Display: image(imread('State.png'))
  Terminator_{1..12} (12 alike) : Terminator
  Trajectories : Subsystem  Tag=Trajectories  mask(PreScan Source Block: Trajectories){}
      mask help:
      | The Trajectory block contains the trajectories defined in the PreScan Experiment Editor. The output of the trajectory block is the (vehicle) State.
      |
      | For more information, please click Help.
      settings: DeleteFcn=PreScanBlockDeleteFcn;
      mask Help: eval('openHelp(312)')
      mask Display: image(imread('Trajectory.png'));
  STATE_Male_RegularAni_1_bus : Outport  Tag=outport/StatePort  OutDataTypeStr=Bus: PRESCAN_STATEACTUATORDATA  PortDimensions=1  SampleTime=1/100
  ANIM_Male_RegularAni_1 : Outport  Tag=outport/AnimationOutport  Port=2  OutDataTypeStr=Bus: PRESCAN_ANIMACTUATORDATA  PortDimensions=1  SampleTime=1/100
  wires:
  STATE_Male_RegularAni_1/1(StateBus) -> STATE_Male_RegularAni_1_bus/1, Animation/1(In1)
  Animation/1(Out1) -> ANIM_Male_RegularAni_1/1
  SELF_Male_RegularAni_1/1 -> SELF_Demux/1(SELF)
  Trajectories/1(State) -> STATE_Male_RegularAni_1/1(State)
  SELF_Demux/1(x [m]) -> Terminator_1/1
  SELF_Demux/2(y [m]) -> Terminator_2/1
  SELF_Demux/3(z [m]) -> Terminator_3/1
  SELF_Demux/4(rotx [deg]) -> Terminator_4/1
  SELF_Demux/5(roty [deg]) -> Terminator_5/1
  SELF_Demux/6(rotz [deg]) -> Terminator_6/1
  SELF_Demux/7(GPS lat [deg]) -> Terminator_7/1
  SELF_Demux/8(GPS long [deg]) -> Terminator_8/1
  SELF_Demux/9(GPS alt [m]) -> Terminator_9/1
  SELF_Demux/10(velocity [m/s]) -> Terminator_10/1
  SELF_Demux/11(heading [deg]) -> Terminator_11/1
  SELF_Demux/12(yaw rate [deg/s]) -> Terminator_12/1

== system Experiment_1_cs/SELF_Actros_2541_1/DISABLED ==
  GND1 : Subsystem
  SELF_Actros_2541_1 : Outport  Tag=outport/SelfPort  OutDataTypeStr=Bus: PRESCAN_SELFSENSORDATA  PortDimensions=1  SampleTime=1/100
  wires:
  GND1/1(bus) -> SELF_Actros_2541_1/1

== system Experiment_1_cs/SELF_Actros_2541_1/ENABLED ==
  Sensor : S-Function  FunctionName=sfun_SelfSensor  Parameters=UniqueID, TimeStep  EnableBusSupport=off  mask(PreScan Source Block: SELF){UniqueID=241, TimeStep=1/100}
      mask prompts: UniqueID "Auto-Assigned: Unique ID"; TimeStep "Auto-Assigned: Upload Period [s]"
      mask help:
      | The SELF port shows (state) information of the actor itself. The outputs are position in the experiment's axis system and the GPS coordinates, and the object's absolute velocity and compass heading.
      |
      | For more information, please click Help.
      mask Help: eval('openHelp(462)')
      mask Display: image(imread('GPS.png'))
  SELF_Actros_2541_1 : Outport  Tag=outport/SelfPort  OutDataTypeStr=Bus: PRESCAN_SELFSENSORDATA  PortDimensions=1  SampleTime=1/100
  wires:
  Sensor/1 -> SELF_Actros_2541_1/1

== system Experiment_1_cs/SELF_Audi_A8_1/DISABLED ==
  GND1 : Subsystem
  SELF_Audi_A8_1 : Outport  Tag=outport/SelfPort  OutDataTypeStr=Bus: PRESCAN_SELFSENSORDATA  PortDimensions=1  SampleTime=1/100
  wires:
  GND1/1(bus) -> SELF_Audi_A8_1/1

== system Experiment_1_cs/SELF_Audi_A8_1/ENABLED ==
  Sensor : S-Function  FunctionName=sfun_SelfSensor  Parameters=UniqueID, TimeStep  EnableBusSupport=off  mask(PreScan Source Block: SELF){UniqueID=256, TimeStep=1/100}
      mask prompts: UniqueID "Auto-Assigned: Unique ID"; TimeStep "Auto-Assigned: Upload Period [s]"
      mask help:
      | The SELF port shows (state) information of the actor itself. The outputs are position in the experiment's axis system and the GPS coordinates, and the object's absolute velocity and compass heading.
      |
      | For more information, please click Help.
      mask Help: eval('openHelp(462)')
      mask Display: image(imread('GPS.png'))
  SELF_Audi_A8_1 : Outport  Tag=outport/SelfPort  OutDataTypeStr=Bus: PRESCAN_SELFSENSORDATA  PortDimensions=1  SampleTime=1/100
  wires:
  Sensor/1 -> SELF_Audi_A8_1/1

== system Experiment_1_cs/SELF_BMW_Z3_1/DISABLED ==
  GND1 : Subsystem
  SELF_BMW_Z3_1 : Outport  Tag=outport/SelfPort  OutDataTypeStr=Bus: PRESCAN_SELFSENSORDATA  PortDimensions=1  SampleTime=1/100
  wires:
  GND1/1(bus) -> SELF_BMW_Z3_1/1

== system Experiment_1_cs/SELF_BMW_Z3_1/ENABLED ==
  Sensor : S-Function  FunctionName=sfun_SelfSensor  Parameters=UniqueID, TimeStep  EnableBusSupport=off  mask(PreScan Source Block: SELF){UniqueID=257, TimeStep=1/100}
      mask prompts: UniqueID "Auto-Assigned: Unique ID"; TimeStep "Auto-Assigned: Upload Period [s]"
      mask help:
      | The SELF port shows (state) information of the actor itself. The outputs are position in the experiment's axis system and the GPS coordinates, and the object's absolute velocity and compass heading.
      |
      | For more information, please click Help.
      mask Help: eval('openHelp(462)')
      mask Display: image(imread('GPS.png'))
  SELF_BMW_Z3_1 : Outport  Tag=outport/SelfPort  OutDataTypeStr=Bus: PRESCAN_SELFSENSORDATA  PortDimensions=1  SampleTime=1/100
  wires:
  Sensor/1 -> SELF_BMW_Z3_1/1

== system Experiment_1_cs/SELF_Male_RegularAni_1/DISABLED ==
  GND1 : Subsystem
  SELF_Male_RegularAni_1 : Outport  Tag=outport/SelfPort  OutDataTypeStr=Bus: PRESCAN_SELFSENSORDATA  PortDimensions=1  SampleTime=1/100
  wires:
  GND1/1(bus) -> SELF_Male_RegularAni_1/1

== system Experiment_1_cs/SELF_Male_RegularAni_1/ENABLED ==
  Sensor : S-Function  FunctionName=sfun_SelfSensor  Parameters=UniqueID, TimeStep  EnableBusSupport=off  mask(PreScan Source Block: SELF){UniqueID=248, TimeStep=1/100}
      mask prompts: UniqueID "Auto-Assigned: Unique ID"; TimeStep "Auto-Assigned: Upload Period [s]"
      mask help:
      | The SELF port shows (state) information of the actor itself. The outputs are position in the experiment's axis system and the GPS coordinates, and the object's absolute velocity and compass heading.
      |
      | For more information, please click Help.
      mask Help: eval('openHelp(462)')
      mask Display: image(imread('GPS.png'))
  SELF_Male_RegularAni_1 : Outport  Tag=outport/SelfPort  OutDataTypeStr=Bus: PRESCAN_SELFSENSORDATA  PortDimensions=1  SampleTime=1/100
  wires:
  Sensor/1 -> SELF_Male_RegularAni_1/1

== system Experiment_1_cs/STATE_Actros_2541_1_bus/DISABLED ==
  STATE_Actros_2541_1_bus : Inport  Tag=inport/StatePort  OutDataTypeStr=Bus: PRESCAN_STATEACTUATORDATA  PortDimensions=1  SampleTime=1/100  BusOutputAsStruct=on
  TRM1 : Terminator
  wires:
  STATE_Actros_2541_1_bus/1 -> TRM1/1

== system Experiment_1_cs/STATE_Actros_2541_1_bus/ENABLED ==
  STATE_Actros_2541_1_bus : Inport  Tag=inport/StatePort  OutDataTypeStr=Bus: PRESCAN_STATEACTUATORDATA  PortDimensions=1  SampleTime=1/100  BusOutputAsStruct=on
  Actuator : S-Function  FunctionName=sfun_StateActuator  Parameters=UniqueID, TimeStep  EnableBusSupport=off  mask(PreScan Sink Block: State){UniqueID=241, TimeStep=1/100}
      mask prompts: UniqueID "Auto-Assigned: Unique ID"; TimeStep "Auto-Assigned: Upload Period [s]"
      mask help:
      | The Actor State contains a vector signal of size (9x1), containing the following signals:
      |
      | -  Position    	(x,y,z)             	[m]
      | -  Velocity    	(vx,vy,vz)         	[m/s]
      | -  Angles       	(Roll, Pitch, Yaw)	[rad]
      |
      | The Actor state is defined in the global axis system.
      | The state is superponed on the Initial position defined in the GUI.
      |
      | For more information, please click Help.
      mask Help: eval('openHelp(222)')
      mask Display: image(imread('State.png'))
  wires:
  STATE_Actros_2541_1_bus/1 -> Actuator/1

== system Experiment_1_cs/STATE_Audi_A8_1_bus/DISABLED ==
  STATE_Audi_A8_1_bus : Inport  Tag=inport/StatePort  OutDataTypeStr=Bus: PRESCAN_STATEACTUATORDATA  PortDimensions=1  SampleTime=1/100  BusOutputAsStruct=on
  TRM1 : Terminator
  wires:
  STATE_Audi_A8_1_bus/1 -> TRM1/1

== system Experiment_1_cs/STATE_Audi_A8_1_bus/ENABLED ==
  STATE_Audi_A8_1_bus : Inport  Tag=inport/StatePort  OutDataTypeStr=Bus: PRESCAN_STATEACTUATORDATA  PortDimensions=1  SampleTime=1/100  BusOutputAsStruct=on
  Actuator : S-Function  FunctionName=sfun_StateActuator  Parameters=UniqueID, TimeStep  EnableBusSupport=off  mask(PreScan Sink Block: State){UniqueID=256, TimeStep=1/100}
      mask prompts: UniqueID "Auto-Assigned: Unique ID"; TimeStep "Auto-Assigned: Upload Period [s]"
      mask help:
      | The Actor State contains a vector signal of size (9x1), containing the following signals:
      |
      | -  Position    	(x,y,z)             	[m]
      | -  Velocity    	(vx,vy,vz)         	[m/s]
      | -  Angles       	(Roll, Pitch, Yaw)	[rad]
      |
      | The Actor state is defined in the global axis system.
      | The state is superponed on the Initial position defined in the GUI.
      |
      | For more information, please click Help.
      mask Help: eval('openHelp(222)')
      mask Display: image(imread('State.png'))
  wires:
  STATE_Audi_A8_1_bus/1 -> Actuator/1

== system Experiment_1_cs/STATE_BMW_Z3_1_bus/DISABLED ==
  STATE_BMW_Z3_1_bus : Inport  Tag=inport/StatePort  OutDataTypeStr=Bus: PRESCAN_STATEACTUATORDATA  PortDimensions=1  SampleTime=1/100  BusOutputAsStruct=on
  TRM1 : Terminator
  wires:
  STATE_BMW_Z3_1_bus/1 -> TRM1/1

== system Experiment_1_cs/STATE_BMW_Z3_1_bus/ENABLED ==
  STATE_BMW_Z3_1_bus : Inport  Tag=inport/StatePort  OutDataTypeStr=Bus: PRESCAN_STATEACTUATORDATA  PortDimensions=1  SampleTime=1/100  BusOutputAsStruct=on
  Actuator : S-Function  FunctionName=sfun_StateActuator  Parameters=UniqueID, TimeStep  EnableBusSupport=off  mask(PreScan Sink Block: State){UniqueID=257, TimeStep=1/100}
      mask prompts: UniqueID "Auto-Assigned: Unique ID"; TimeStep "Auto-Assigned: Upload Period [s]"
      mask help:
      | The Actor State contains a vector signal of size (9x1), containing the following signals:
      |
      | -  Position    	(x,y,z)             	[m]
      | -  Velocity    	(vx,vy,vz)         	[m/s]
      | -  Angles       	(Roll, Pitch, Yaw)	[rad]
      |
      | The Actor state is defined in the global axis system.
      | The state is superponed on the Initial position defined in the GUI.
      |
      | For more information, please click Help.
      mask Help: eval('openHelp(222)')
      mask Display: image(imread('State.png'))
  wires:
  STATE_BMW_Z3_1_bus/1 -> Actuator/1

== system Experiment_1_cs/STATE_Male_RegularAni_1_bus/DISABLED ==
  STATE_Male_RegularAni_1_bus : Inport  Tag=inport/StatePort  OutDataTypeStr=Bus: PRESCAN_STATEACTUATORDATA  PortDimensions=1  SampleTime=1/100  BusOutputAsStruct=on
  TRM1 : Terminator
  wires:
  STATE_Male_RegularAni_1_bus/1 -> TRM1/1

== system Experiment_1_cs/STATE_Male_RegularAni_1_bus/ENABLED ==
  STATE_Male_RegularAni_1_bus : Inport  Tag=inport/StatePort  OutDataTypeStr=Bus: PRESCAN_STATEACTUATORDATA  PortDimensions=1  SampleTime=1/100  BusOutputAsStruct=on
  Actuator : S-Function  FunctionName=sfun_StateActuator  Parameters=UniqueID, TimeStep  EnableBusSupport=off  mask(PreScan Sink Block: State){UniqueID=248, TimeStep=1/100}
      mask prompts: UniqueID "Auto-Assigned: Unique ID"; TimeStep "Auto-Assigned: Upload Period [s]"
      mask help:
      | The Actor State contains a vector signal of size (9x1), containing the following signals:
      |
      | -  Position    	(x,y,z)             	[m]
      | -  Velocity    	(vx,vy,vz)         	[m/s]
      | -  Angles       	(Roll, Pitch, Yaw)	[rad]
      |
      | The Actor state is defined in the global axis system.
      | The state is superponed on the Initial position defined in the GUI.
      |
      | For more information, please click Help.
      mask Help: eval('openHelp(222)')
      mask Display: image(imread('State.png'))
  wires:
  STATE_Male_RegularAni_1_bus/1 -> Actuator/1

== system Experiment_1_cs/TIS_1/DISABLED ==
  GND1 : Subsystem
  TIS_1 : Outport  Tag=outport/TIS  OutDataTypeStr=Bus: PRESCAN_SCANNERSENSOR_MESSAGE  PortDimensions=1  SampleTime=1/50
  wires:
  GND1/1(bus) -> TIS_1/1

== system Experiment_1_cs/TIS_1/ENABLED ==
  Sensor : S-Function  FunctionName=sfun_TIS  Parameters=sensorID, detectableObjects, timestep  EnableBusSupport=off  mask(PreScan Source Block: Technology Independent Sensor (TIS)){sensorID=258, detectableObjects=1, timestep=1/50}
      mask prompts: sensorID "Sensor ID"; detectableObjects "Max detectable objects:"; timestep "MATLAB timestep:"
      mask help:
      | The Technology Independent Sensor (TIS) provides a sensor with all sensor-related influence factors (like noise, drift and accuracy) without being technology specific (like radar and lidar). The TIS detects the closest point on the geometry of an object.
      |
      | For more information, please click Help.
      mask Help: eval('openHelp(449)')
      mask Display: image(imread('TIS.png'))
  TIS_1 : Outport  Tag=outport/TIS  OutDataTypeStr=Bus: PRESCAN_SCANNERSENSOR_MESSAGE  PortDimensions=1  SampleTime=1/50
  wires:
  Sensor/1 -> TIS_1/1

== system Experiment_1_cs/TIS_2/DISABLED ==
  GND1 : Subsystem
  TIS_2 : Outport  Tag=outport/TIS  OutDataTypeStr=Bus: PRESCAN_SCANNERSENSOR_MESSAGE  PortDimensions=1  SampleTime=1/50
  wires:
  GND1/1(bus) -> TIS_2/1

== system Experiment_1_cs/TIS_2/ENABLED ==
  Sensor : S-Function  FunctionName=sfun_TIS  Parameters=sensorID, detectableObjects, timestep  EnableBusSupport=off  mask(PreScan Source Block: Technology Independent Sensor (TIS)){sensorID=263, detectableObjects=1, timestep=1/50}
      mask prompts: sensorID "Sensor ID"; detectableObjects "Max detectable objects:"; timestep "MATLAB timestep:"
      mask help:
      | The Technology Independent Sensor (TIS) provides a sensor with all sensor-related influence factors (like noise, drift and accuracy) without being technology specific (like radar and lidar). The TIS detects the closest point on the geometry of an object.
      |
      | For more information, please click Help.
      mask Help: eval('openHelp(449)')
      mask Display: image(imread('TIS.png'))
  TIS_2 : Outport  Tag=outport/TIS  OutDataTypeStr=Bus: PRESCAN_SCANNERSENSOR_MESSAGE  PortDimensions=1  SampleTime=1/50
  wires:
  Sensor/1 -> TIS_2/1

== system Experiment_1_cs/V2X_Rx262_Generic_Receiver/DISABLED ==
  GND1 : Ground
  V2X_Rx262_Generic_Receiver : Outport  Tag=outport/plugin/sfun_V2X_Generic_Receiver
  wires:
  GND1/1 -> V2X_Rx262_Generic_Receiver/1

== system Experiment_1_cs/V2X_Rx262_Generic_Receiver/ENABLED ==
  Sensor : S-Function  LoadFcn=load('Generic.mat');  FunctionName=sfun_V2X_Generic_Receiver  Parameters=sensorID, parentID, maxMessages, timestep  EnableBusSupport=off  mask(V2X Generic Receiver Block){sensorID=262, parentID=256, maxMessages=1, timestep=1/100}
      mask prompts: sensorID "Receiver ID"; parentID "Parent ID"; maxMessages "Maximum number of messages"; timestep "MATLAB timestep:"
      mask help: V2X Block receiving a Generic message
      mask Display: image(imread('V2XR_grayscale.png'))
  V2X_Rx262_Generic_Receiver : Outport  Tag=outport/plugin/sfun_V2X_Generic_Receiver
  wires:
  Sensor/1 -> V2X_Rx262_Generic_Receiver/1

== system Experiment_1_cs/V2X_Rx264_Generic_Receiver/DISABLED ==
  GND1 : Ground
  V2X_Rx264_Generic_Receiver : Outport  Tag=outport/plugin/sfun_V2X_Generic_Receiver
  wires:
  GND1/1 -> V2X_Rx264_Generic_Receiver/1

== system Experiment_1_cs/V2X_Rx264_Generic_Receiver/ENABLED ==
  Sensor : S-Function  LoadFcn=load('Generic.mat');  FunctionName=sfun_V2X_Generic_Receiver  Parameters=sensorID, parentID, maxMessages, timestep  EnableBusSupport=off  mask(V2X Generic Receiver Block){sensorID=264, parentID=257, maxMessages=1, timestep=1/100}
      mask prompts: sensorID "Receiver ID"; parentID "Parent ID"; maxMessages "Maximum number of messages"; timestep "MATLAB timestep:"
      mask help: V2X Block receiving a Generic message
      mask Display: image(imread('V2XR_grayscale.png'))
  V2X_Rx264_Generic_Receiver : Outport  Tag=outport/plugin/sfun_V2X_Generic_Receiver
  wires:
  Sensor/1 -> V2X_Rx264_Generic_Receiver/1

== system Experiment_1_cs/V2X_Tx262_Generic_Transmitter/DISABLED ==
  V2X_Tx262_Generic_Transmitter : Inport  Tag=inport/plugin/sfun_V2X_Generic_Transmitter  BusOutputAsStruct=on
  TRM1 : Terminator
  wires:
  V2X_Tx262_Generic_Transmitter/1 -> TRM1/1

== system Experiment_1_cs/V2X_Tx262_Generic_Transmitter/ENABLED ==
  V2X_Tx262_Generic_Transmitter : Inport  Tag=inport/plugin/sfun_V2X_Generic_Transmitter  BusOutputAsStruct=on
  Actuator : S-Function  LoadFcn=load('Generic.mat');  FunctionName=sfun_V2X_Generic_Transmitter  Parameters=sensorID, parentID, timestep  EnableBusSupport=off  mask(V2X Generic Transmitter Block){sensorID=262, parentID=256, timestep=1/100}
      mask prompts: sensorID "Transmitter ID"; parentID "Parent ID"; timestep "MATLAB timestep:"
      mask help: V2X Block transmitting a Generic message
      mask Display: image(imread('V2XT_grayscale.png'))
  wires:
  V2X_Tx262_Generic_Transmitter/1 -> Actuator/1

== system Experiment_1_cs/V2X_Tx264_Generic_Transmitter/DISABLED ==
  V2X_Tx264_Generic_Transmitter : Inport  Tag=inport/plugin/sfun_V2X_Generic_Transmitter  BusOutputAsStruct=on
  TRM1 : Terminator
  wires:
  V2X_Tx264_Generic_Transmitter/1 -> TRM1/1

== system Experiment_1_cs/V2X_Tx264_Generic_Transmitter/ENABLED ==
  V2X_Tx264_Generic_Transmitter : Inport  Tag=inport/plugin/sfun_V2X_Generic_Transmitter  BusOutputAsStruct=on
  Actuator : S-Function  LoadFcn=load('Generic.mat');  FunctionName=sfun_V2X_Generic_Transmitter  Parameters=sensorID, parentID, timestep  EnableBusSupport=off  mask(V2X Generic Transmitter Block){sensorID=264, parentID=257, timestep=1/100}
      mask prompts: sensorID "Transmitter ID"; parentID "Parent ID"; timestep "MATLAB timestep:"
      mask help: V2X Block transmitting a Generic message
      mask Display: image(imread('V2XT_grayscale.png'))
  wires:
  V2X_Tx264_Generic_Transmitter/1 -> Actuator/1

== system Experiment_1_cs/Actros_2541_1/DISABLED/GND1 ==
  GND_AccelerationX : Constant  Value=0
  GND_AccelerationY : Constant  Value=0
  GND_AccelerationZ : Constant  Value=0
  GND_AngularVelocityPitch : Constant  Value=0
  GND_AngularVelocityRoll : Constant  Value=0
  GND_AngularVelocityYaw : Constant  Value=0
  GND_OrientationPitch : Constant  Value=0
  GND_OrientationRoll : Constant  Value=0
  GND_OrientationYaw : Constant  Value=0
  GND_PositionX : Constant  Value=0
  GND_PositionY : Constant  Value=0
  GND_PositionZ : Constant  Value=0
  GND_VelocityX : Constant  Value=0
  GND_VelocityY : Constant  Value=0
  GND_VelocityZ : Constant  Value=0
  buscreator : BusCreator  Inputs=15  OutDataTypeStr=Bus: PRESCAN_STATEACTUATORDATA  NonVirtualBus=on
  bus : Outport  OutDataTypeStr=Bus: PRESCAN_STATEACTUATORDATA
  wires:
  GND_PositionX/1 -> buscreator/1  "PositionX"
  GND_PositionY/1 -> buscreator/2  "PositionY"
  GND_PositionZ/1 -> buscreator/3  "PositionZ"
  GND_VelocityX/1 -> buscreator/4  "VelocityX"
  GND_VelocityY/1 -> buscreator/5  "VelocityY"
  GND_VelocityZ/1 -> buscreator/6  "VelocityZ"
  GND_AccelerationX/1 -> buscreator/7  "AccelerationX"
  GND_AccelerationY/1 -> buscreator/8  "AccelerationY"
  GND_AccelerationZ/1 -> buscreator/9  "AccelerationZ"
  GND_OrientationRoll/1 -> buscreator/10  "OrientationRoll"
  GND_OrientationPitch/1 -> buscreator/11  "OrientationPitch"
  GND_OrientationYaw/1 -> buscreator/12  "OrientationYaw"
  GND_AngularVelocityRoll/1 -> buscreator/13  "AngularVelocityRoll"
  GND_AngularVelocityPitch/1 -> buscreator/14  "AngularVelocityPitch"
  GND_AngularVelocityYaw/1 -> buscreator/15  "AngularVelocityYaw"
  buscreator/1 -> bus/1

== system Experiment_1_cs/Actros_2541_1/ENABLED/Dynamics_Empty ==
  note: For state mode 'Dynamic' positions
      | are not taken into account, as they
      | are computed by integrating velocity.
      | Click annotation for Help.
  Ground_{1..9} (9 alike) : Ground
  MuxState : Subsystem  Tag=mux/State  mask(Empty Dynamics State Block){positioningmode=on, TimeStep=1/100}
      mask prompts: positioningmode "Positioning Mode"; TimeStep "Auto Assigned: Time Step [s]"
      mask help:
      | Build the state of an actor based on user input.
      | The user can either use positioning mode or dynamics mode.
      | - When using positioning mode the position and orientation of the actor are set directly based on the input. Expected input is relative to the initial position and orientation of the actor. It's also possible to specify the velocity of the actor, though this input isn't used, only passed on.
      | - When using dynamics mode the position input is ignored. Expected input is velocity and orientation. The velocity is relative the current orientation of the actor, while orientation is relative to its initial orientation. The position of the actor is calculated based on the velocity and orientation given.
      settings: DeleteFcn=PreScanBlockDeleteFcn;
  State : Outport  Tag=outport/StateOutport  SampleTime=1/100
  wires:
  MuxState/1(state) -> State/1
  Ground_1/1 -> MuxState/1(x [m])
  Ground_2/1 -> MuxState/2(y [m])
  Ground_3/1 -> MuxState/3(z [m])
  Ground_4/1 -> MuxState/4(dx [m/s])
  Ground_5/1 -> MuxState/5(dy [m/s])
  Ground_6/1 -> MuxState/6(dz [m/s])
  Ground_7/1 -> MuxState/7(R [rad])
  Ground_8/1 -> MuxState/8(P [rad])
  Ground_9/1 -> MuxState/9(Y [rad])
